simulink model "SACLaunch"  (R2019b)
settings: Solver=FixedStepDiscrete  StartTime=0  StopTime=1452  RelTol=1e-3
undefined symbols (not defined in the file or in its folder): DiscIntNeverNeededParam
libraries: simulink x1
settings Model: Creator=user  LastModifiedBy=yuxia

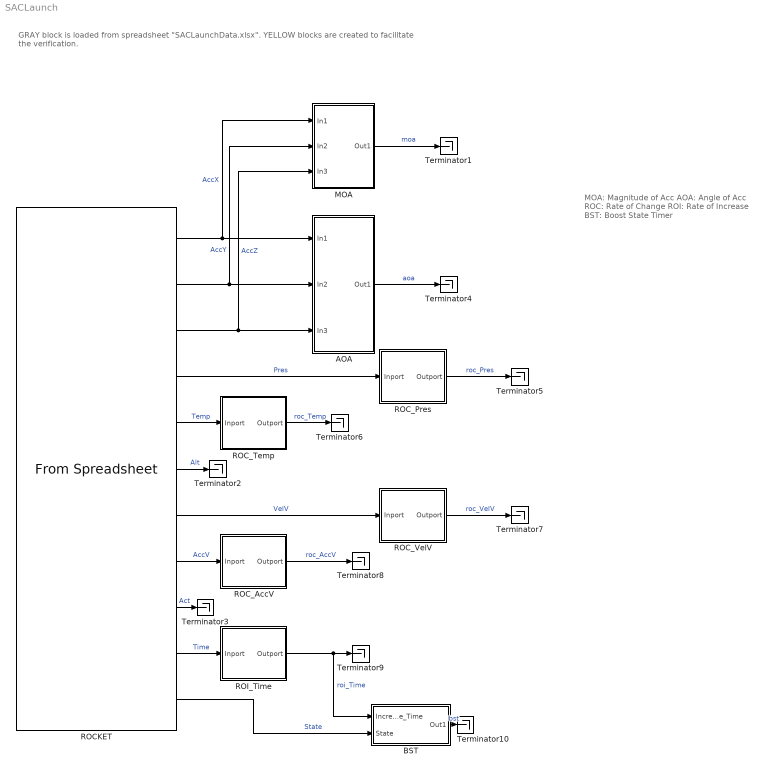
== system SACLaunch ==
  note: MOA: Magnitude of Acc
      | AOA: Angle of Acc
      | ROC: Rate of Change
      | ROI: Rate of Increase
      | BST: Boost State Timer
  note: GRAY block is loaded from spreadsheet "SACLaunchData.xlsx".
      | YELLOW blocks are created to facilitate the verification.
  AOA : Subsystem
  BST : Subsystem
  MOA : Subsystem
  ROCKET : FromSpreadsheet  Tag=NovaSomniumRocket  FileName=SACLaunchData.xlsx  SheetName=SACLaunchData  SampleTime=0.001  ExtrapolationBeforeFirstDataPoint=Ground value  InterpolationWithinTimeRange=Zero order hold  ExtrapolationAfterLastDataPoint=Ground value
  ROC_AccV : Subsystem
      mask Display: set_param(gcb,'BackgroundColor','yellow');
  ROC_Pres : Subsystem
      mask Display: set_param(gcb,'BackgroundColor','yellow');
  ROC_Temp : Subsystem
      mask Display: set_param(gcb,'BackgroundColor','yellow');
  ROC_VelV : Subsystem
      mask Display: set_param(gcb,'BackgroundColor','yellow');
  ROI_Time : Subsystem
      mask Display: set_param(gcb,'BackgroundColor','yellow');
  Terminator{1..10} (10 alike) : Terminator
  wires:
  ROCKET/4 -> ROC_Pres/1(Inport)  "Pres"
  ROCKET/6 -> Terminator2/1  "Alt"
  ROCKET/8 -> ROC_AccV/1(Inport)  "AccV"
  ROCKET/10 -> ROI_Time/1(Inport)  "Time"
  AOA/1(Out1) -> Terminator4/1  "aoa"
  ROCKET/5 -> ROC_Temp/1(Inport)  "Temp"
  ROC_Temp/1(Outport) -> Terminator6/1  "roc_Temp"
  ROC_Pres/1(Outport) -> Terminator5/1  "roc_Pres"
  ROC_AccV/1(Outport) -> Terminator8/1  "roc_AccV"
  ROI_Time/1(Outport) -> Terminator9/1, BST/1(Increase_Time)  "roi_Time"
  ROCKET/7 -> ROC_VelV/1(Inport)  "VelV"
  ROC_VelV/1(Outport) -> Terminator7/1  "roc_VelV"
  ROCKET/9 -> Terminator3/1  "Act"
  ROCKET/1 -> MOA/1(In1), AOA/1(In1)  "AccX"
  ROCKET/2 -> MOA/2(In2), AOA/2(In2)  "AccY"
  ROCKET/3 -> MOA/3(In3), AOA/3(In3)  "AccZ"
  MOA/1(Out1) -> Terminator1/1  "moa"
  ROCKET/11 -> BST/2(State)  "State"
  BST/1(Out1) -> Terminator10/1  "bst"

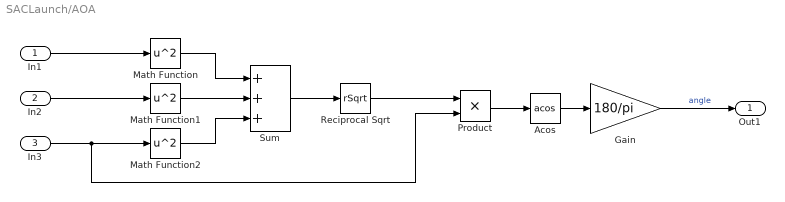
== system SACLaunch/AOA ==
  In1 : Inport
  In2 : Inport  Port=2
  In3 : Inport  Port=3
  Acos : Trigonometry  Operator=acos
  Gain : Gain  Gain=180/pi
  Math Function : Math  Operator=square  SignedPower=off  SaturateOnIntegerOverflow=on
  Math Function1 : Math  Operator=square  SignedPower=off  SaturateOnIntegerOverflow=on
  Math Function2 : Math  Operator=square  SignedPower=off  SaturateOnIntegerOverflow=on
  Product : Product
  Reciprocal Sqrt : Sqrt  Operator=rSqrt  SaturateOnIntegerOverflow=on
  Sum : Sum  Inputs=+++
  Out1 : Outport
  wires:
  Math Function1/1 -> Sum/2
  Acos/1 -> Gain/1
  Sum/1 -> Reciprocal Sqrt/1
  In2/1 -> Math Function1/1
  In3/1 -> Product/2, Math Function2/1
  Product/1 -> Acos/1
  Gain/1 -> Out1/1  "angle"
  Math Function/1 -> Sum/1
  Reciprocal Sqrt/1 -> Product/1
  In1/1 -> Math Function/1
  Math Function2/1 -> Sum/3

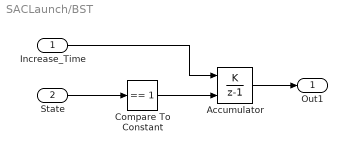
== system SACLaunch/BST ==
  Increase_Time : Inport
  State : Inport  Port=2
  Accumulator : DiscreteIntegrator  IntegratorMethod=Accumulation: Forward Euler  ExternalReset=rising  SampleTime=-1  ICPrevOutput=DiscIntNeverNeededParam  ICPrevScaledInput=DiscIntNeverNeededParam
  Compare To Constant : simulink/Logic and Bit Operations/Compare To Constant  relop===  const=1  OutDataTypeStr=boolean
  Out1 : Outport
  wires:
  Increase_Time/1 -> Accumulator/1
  State/1 -> Compare To Constant/1
  Compare To Constant/1 -> Accumulator/2
  Accumulator/1 -> Out1/1

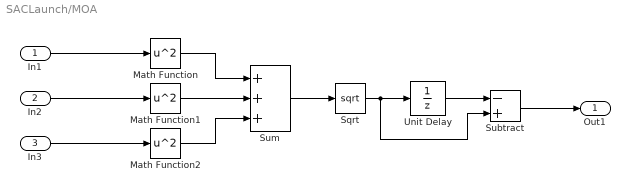
== system SACLaunch/MOA ==
  In1 : Inport
  In2 : Inport  Port=2
  In3 : Inport  Port=3
  Math Function : Math  Operator=square  SignedPower=off  SaturateOnIntegerOverflow=on
  Math Function1 : Math  Operator=square  SignedPower=off  SaturateOnIntegerOverflow=on
  Math Function2 : Math  Operator=square  SignedPower=off  SaturateOnIntegerOverflow=on
  Sqrt : Sqrt  SaturateOnIntegerOverflow=on
  Subtract : Sum  Inputs=-+
  Sum : Sum  Inputs=+++
  Unit Delay : UnitDelay  SampleTime=-1  HasFrameUpgradeWarning=on
  Out1 : Outport
  wires:
  Math Function2/1 -> Sum/3
  Math Function/1 -> Sum/1
  Unit Delay/1 -> Subtract/1
  Sum/1 -> Sqrt/1
  In3/1 -> Math Function2/1
  Sqrt/1 -> Subtract/2, Unit Delay/1
  Math Function1/1 -> Sum/2
  In2/1 -> Math Function1/1
  In1/1 -> Math Function/1
  Subtract/1 -> Out1/1

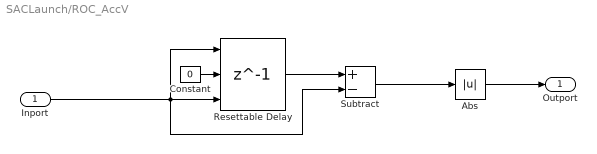
== system SACLaunch/ROC_AccV ==
  Inport : Inport
  Abs : Abs
  Constant : Constant  Value=0
  Resettable Delay : Delay  DelayLength=1  InitialConditionSource=Input port  ExternalReset=Rising
      settings: InputPortMap=u0,r5,p4
  Subtract : Sum  Inputs=+-
  Outport : Outport
  wires:
  Subtract/1 -> Abs/1
  Inport/1 -> Subtract/2, Resettable Delay/3, Resettable Delay/1
  Resettable Delay/1 -> Subtract/1
  Constant/1 -> Resettable Delay/2
  Abs/1 -> Outport/1

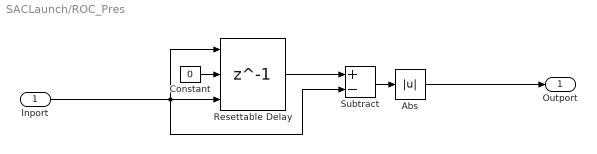
== system SACLaunch/ROC_Pres ==
  Inport : Inport
  Abs : Abs
  Constant : Constant  Value=0
  Resettable Delay : Delay  DelayLength=1  InitialConditionSource=Input port  ExternalReset=Rising
      settings: InputPortMap=u0,r5,p4
  Subtract : Sum  Inputs=+-
  Outport : Outport
  wires:
  Subtract/1 -> Abs/1
  Inport/1 -> Subtract/2, Resettable Delay/3, Resettable Delay/1
  Resettable Delay/1 -> Subtract/1
  Constant/1 -> Resettable Delay/2
  Abs/1 -> Outport/1

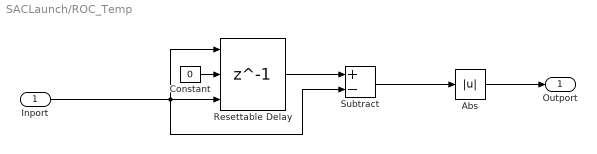
== system SACLaunch/ROC_Temp ==
  Inport : Inport
  Abs : Abs
  Constant : Constant  Value=0
  Resettable Delay : Delay  DelayLength=1  InitialConditionSource=Input port  ExternalReset=Rising
      settings: InputPortMap=u0,r5,p4
  Subtract : Sum  Inputs=+-
  Outport : Outport
  wires:
  Subtract/1 -> Abs/1
  Inport/1 -> Subtract/2, Resettable Delay/3, Resettable Delay/1
  Resettable Delay/1 -> Subtract/1
  Constant/1 -> Resettable Delay/2
  Abs/1 -> Outport/1

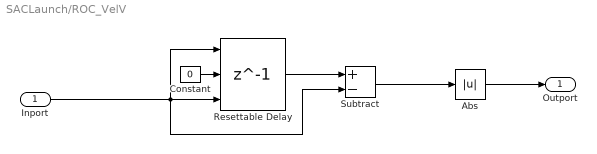
== system SACLaunch/ROC_VelV ==
  Inport : Inport
  Abs : Abs
  Constant : Constant  Value=0
  Resettable Delay : Delay  DelayLength=1  InitialConditionSource=Input port  ExternalReset=Rising
      settings: InputPortMap=u0,r5,p4
  Subtract : Sum  Inputs=+-
  Outport : Outport
  wires:
  Subtract/1 -> Abs/1
  Inport/1 -> Subtract/2, Resettable Delay/3, Resettable Delay/1
  Resettable Delay/1 -> Subtract/1
  Constant/1 -> Resettable Delay/2
  Abs/1 -> Outport/1

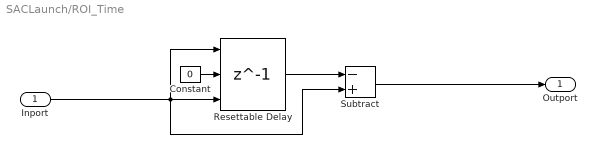
== system SACLaunch/ROI_Time ==
  Inport : Inport
  Constant : Constant  Value=0
  Resettable Delay : Delay  DelayLength=1  InitialConditionSource=Input port  ExternalReset=Rising
      settings: InputPortMap=u0,r5,p4
  Subtract : Sum  Inputs=-+
  Outport : Outport
  wires:
  Inport/1 -> Subtract/2, Resettable Delay/3, Resettable Delay/1
  Resettable Delay/1 -> Subtract/1
  Constant/1 -> Resettable Delay/2
  Subtract/1 -> Outport/1
